simulink model "q"  (R2017b)
settings: Solver=ode5  StartTime=0.0  StopTime=10.0  FixedStep=60  RelTol=1e-3
values from neighbouring files (symbols this model uses):
  AU = 1.496e11    (= 149600000000)    [Dyn_kin.m]    (also in trans_kin_dyn.m)
  c = SC.Polyhedron.C    [Dyn_kin.m]    (also in trans_kin_dyn.m)
  G = 6.674080000000000e-11    (= 6.67408e-11)    [Dyn_kin.m]    (also in trans_kin_dyn.m)
  mu_s = 1.326807104e20    (= 1.326807104e+20)    [Dyn_kin.m]    (also in trans_kin_dyn.m)
  T = [0 2000]    [Att_dyn.m]    (also in Att_kin.m; Dyn_kin.m = [0 1000]; trans_kin_dyn.m = [0 1000])
undefined symbols (not defined in the file or in its folder): bias, Cube, K_d, K_p, noise, P_k0, SC, std_noise, Sun, x_k0
settings Model: Creator=hazr_sh  LastModifiedBy=hazr_sh

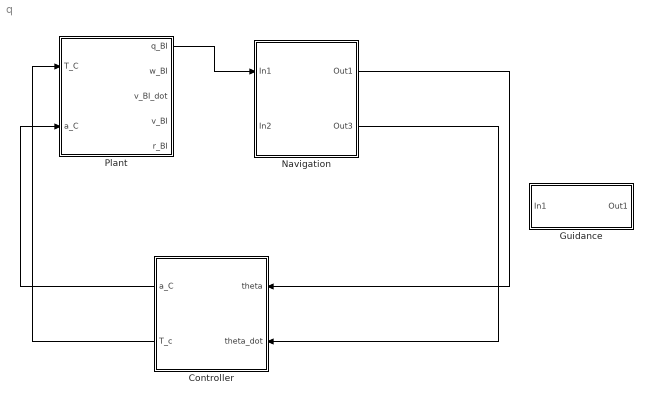
== system q ==
  Controller : Subsystem
  Guidance : Subsystem
  Navigation : Subsystem
  Plant : Subsystem
  wires:
  Controller/2(T_c) -> Plant/1(T_C)
  Plant/1(q_BI) -> Navigation/1(In1)
  ? -> Navigation/2(In2)
  Navigation/1(Out1) -> Controller/1(theta)
  Navigation/2(Out3) -> Controller/2(theta_dot)
  Controller/1(a_C) -> Plant/2(a_C)

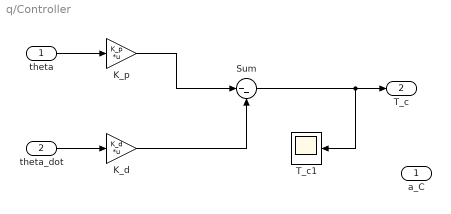
== system q/Controller ==
  theta : Inport
  theta_dot : Inport  Port=2
  K_d : Gain  Gain=K_d  Multiplication=Matrix(K*u)
  K_p : Gain  Gain=K_p  Multiplication=Matrix(K*u)
  Sum : Sum  Inputs=|--
  T_c1 : Scope
  a_C : Outport
  T_c : Outport  Port=2
  wires:
  theta_dot/1 -> K_d/1
  theta/1 -> K_p/1
  K_p/1 -> Sum/1
  K_d/1 -> Sum/2
  Sum/1 -> T_c1/1, T_c/1

== system q/Guidance ==
  In1 : Inport
  Out1 : Outport
  wires:
  In1/1 -> Out1/1

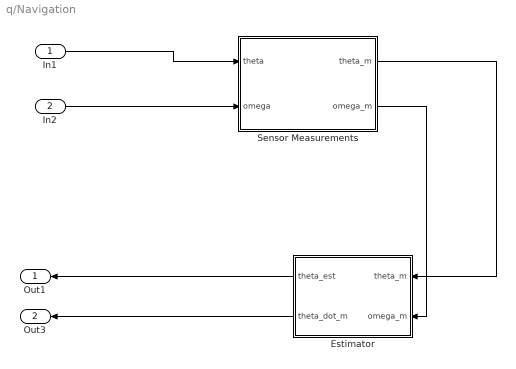
== system q/Navigation ==
  In1 : Inport
  In2 : Inport  Port=2
  Estimator : Subsystem
  Sensor Measurements : Subsystem
  Out1 : Outport
  Out3 : Outport  Port=2
  wires:
  Sensor Measurements/2(omega_m) -> Estimator/2(omega_m)
  In2/1 -> Sensor Measurements/2(omega)
  Estimator/1(theta_est) -> Out1/1
  Estimator/2(theta_dot_m) -> Out3/1
  Sensor Measurements/1(theta_m) -> Estimator/1(theta_m)
  In1/1 -> Sensor Measurements/1(theta)

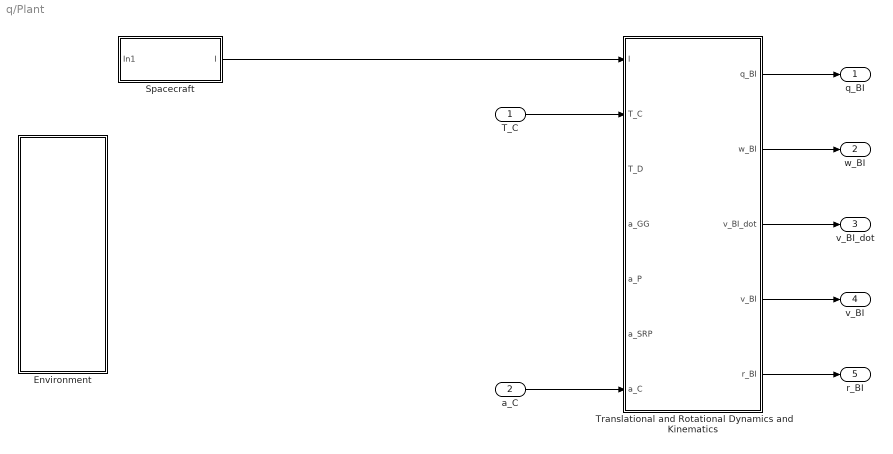
== system q/Plant ==
  T_C : Inport
  a_C : Inport  Port=2
  Environment : Subsystem
  Spacecraft : Subsystem
  Translational and Rotational Dynamics and Kinematics : Subsystem
  q_BI : Outport
  w_BI : Outport  Port=2
  v_BI_dot : Outport  Port=3
  v_BI : Outport  Port=4
  r_BI : Outport  Port=5
  wires:
  Translational and Rotational Dynamics and Kinematics/1(q_BI) -> q_BI/1
  Translational and Rotational Dynamics and Kinematics/2(w_BI) -> w_BI/1
  Translational and Rotational Dynamics and Kinematics/3(v_BI_dot) -> v_BI_dot/1
  Translational and Rotational Dynamics and Kinematics/4(v_BI) -> v_BI/1
  Translational and Rotational Dynamics and Kinematics/5(r_BI) -> r_BI/1
  ? -> Translational and Rotational Dynamics and Kinematics/4(a_GG)
  ? -> Translational and Rotational Dynamics and Kinematics/5(a_P)
  ? -> Translational and Rotational Dynamics and Kinematics/6(a_SRP)
  a_C/1 -> Translational and Rotational Dynamics and Kinematics/7(a_C)
  T_C/1 -> Translational and Rotational Dynamics and Kinematics/2(T_C)
  Spacecraft/1(I) -> Translational and Rotational Dynamics and Kinematics/1(I)
  ? -> Translational and Rotational Dynamics and Kinematics/3(T_D)

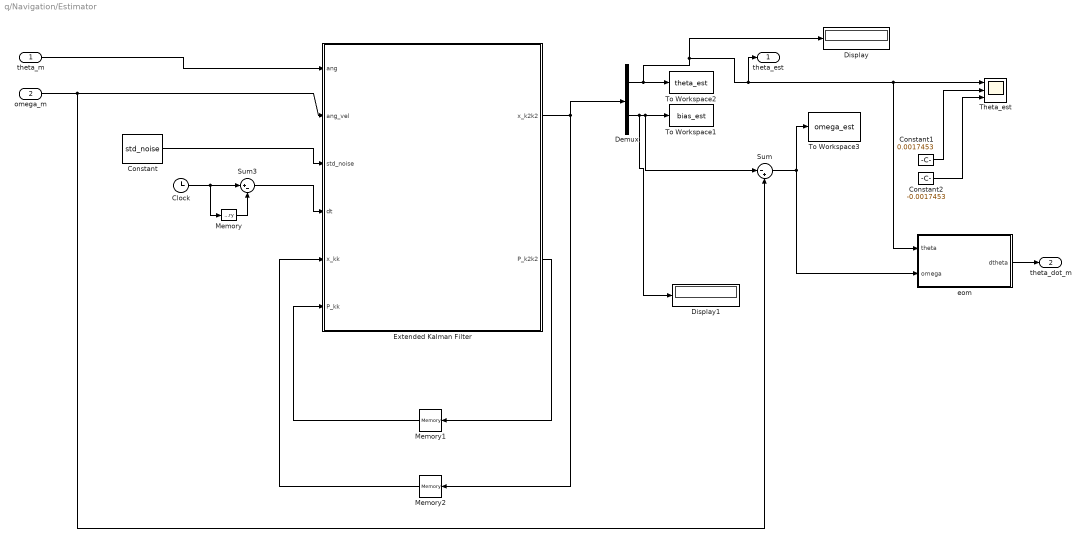
== system q/Navigation/Estimator ==
  theta_m : Inport
  omega_m : Inport  Port=2
  " Extended Kalman Filter" : MATLAB Function  TreatAsAtomicUnit=on
  Clock : Clock
  Constant : Constant  Value=std_noise  VectorParams1D=off
  Constant1 : Constant  Value=0.0017453
  Constant2 : Constant  Value=-0.0017453
  Demux : Demux  Outputs=2
  Display : Display
  Display1 : Display
  Memory : Memory
  Memory1 : Memory  InitialCondition=P_k0
  Memory2 : Memory  InitialCondition=x_k0
  Sum : Sum  Inputs=|-+
  Sum3 : Sum  Inputs=|+-
  Theta_est : Scope  NumInputPorts=3
  To Workspace1 : ToWorkspace  VariableName=bias_est  SampleTime=-1
  To Workspace2 : ToWorkspace  VariableName=theta_est  SampleTime=-1
  To Workspace3 : ToWorkspace  VariableName=omega_est  SampleTime=-1
  "eom " : MATLAB Function  TreatAsAtomicUnit=on
  theta_est : Outport
  theta_dot_m : Outport  Port=2
  wires:
  Memory1/1 -> " Extended Kalman Filter"/6(P_kk)
  theta_m/1 -> " Extended Kalman Filter"/1(ang)
  Memory/1 -> Sum3/2
  Clock/1 -> Memory/1, Sum3/1
  " Extended Kalman Filter"/2(P_k2k2) -> Memory1/1
  " Extended Kalman Filter"/1(x_k2k2) -> Demux/1, Memory2/1
  Sum3/1 -> " Extended Kalman Filter"/4(dt)
  omega_m/1 -> Sum/2, " Extended Kalman Filter"/2(ang_vel)
  Memory2/1 -> " Extended Kalman Filter"/5(x_kk)
  Constant/1 -> " Extended Kalman Filter"/3(std_noise)
  Constant1/1 -> Theta_est/2
  Constant2/1 -> Theta_est/3
  Sum/1 -> To Workspace3/1, "eom "/2(omega)
  "eom "/1(dtheta) -> theta_dot_m/1
  Demux/1 -> To Workspace2/1, theta_est/1, "eom "/1(theta), Theta_est/1, Display/1
  Demux/2 -> Sum/1, To Workspace1/1, Display1/1

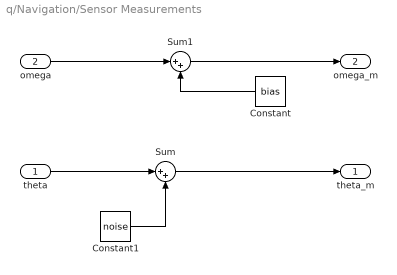
== system q/Navigation/Sensor Measurements ==
  theta : Inport
  omega : Inport  Port=2
  Constant : Constant  Value=bias  VectorParams1D=off
  Constant1 : Constant  Value=noise  VectorParams1D=off
  Sum : Sum  Inputs=|++
  Sum1 : Sum  Inputs=|++
  theta_m : Outport
  omega_m : Outport  Port=2
  wires:
  theta/1 -> Sum/1
  Constant1/1 -> Sum/2
  omega/1 -> Sum1/1
  Constant/1 -> Sum1/2
  Sum/1 -> theta_m/1
  Sum1/1 -> omega_m/1

== system q/Plant/Environment ==
  Asteroid Kinematics and Dynamics : Subsystem
  Disturbances : Subsystem

== system q/Plant/Spacecraft ==
  In1 : Inport
  Switch : Switch  Criteria=u2 > Threshold
  I : Outport
  wires:
  In1/1 -> I/1

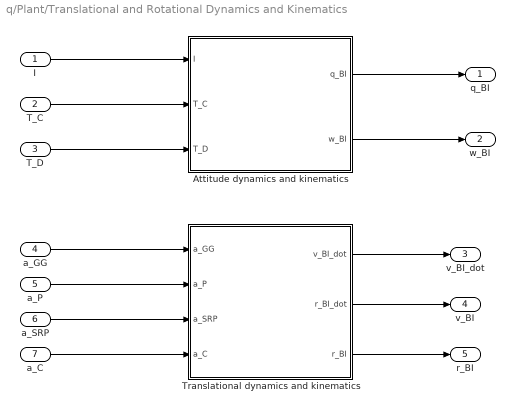
== system q/Plant/Translational and Rotational Dynamics and Kinematics ==
  I : Inport
  T_C : Inport  Port=2
  T_D : Inport  Port=3
  a_GG : Inport  Port=4
  a_P : Inport  Port=5
  a_SRP : Inport  Port=6
  a_C : Inport  Port=7
  Attitude dynamics and kinematics : Subsystem
  Translational dynamics and kinematics : Subsystem
  q_BI : Outport
  w_BI : Outport  Port=2
  v_BI_dot : Outport  Port=3
  v_BI : Outport  Port=4
  r_BI : Outport  Port=5
  wires:
  T_D/1 -> Attitude dynamics and kinematics/3(T_D)
  a_GG/1 -> Translational dynamics and kinematics/1(a_GG)
  a_SRP/1 -> Translational dynamics and kinematics/3(a_SRP)
  a_P/1 -> Translational dynamics and kinematics/2(a_P)
  I/1 -> Attitude dynamics and kinematics/1(I)
  Translational dynamics and kinematics/2(r_BI_dot) -> v_BI/1
  Attitude dynamics and kinematics/1(q_BI) -> q_BI/1
  T_C/1 -> Attitude dynamics and kinematics/2(T_C)
  Translational dynamics and kinematics/3(r_BI) -> r_BI/1
  Translational dynamics and kinematics/1(v_BI_dot) -> v_BI_dot/1
  Attitude dynamics and kinematics/2(w_BI) -> w_BI/1
  a_C/1 -> Translational dynamics and kinematics/4(a_C)

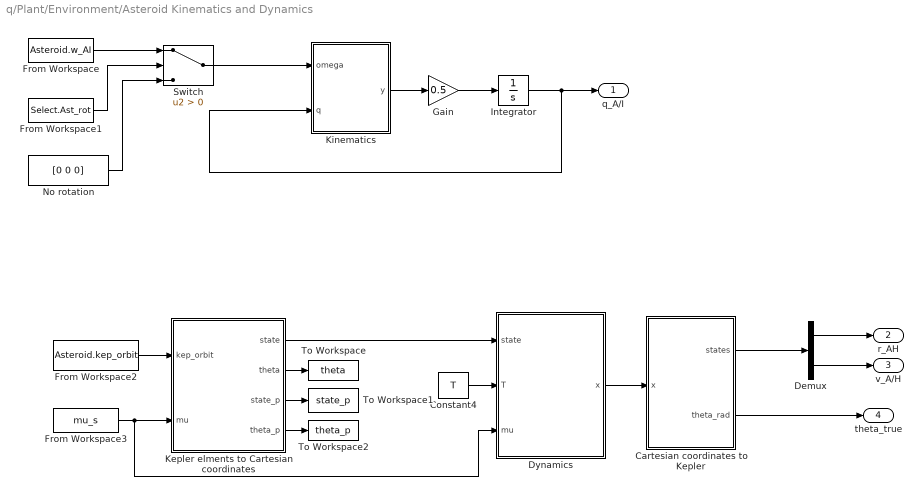
== system q/Plant/Environment/Asteroid Kinematics and Dynamics ==
  Cartesian coordinates to Kepler : MATLAB Function  TreatAsAtomicUnit=on
  Constant4 : Constant  Value=T
  Demux : Demux  Outputs=2
  Dynamics : MATLAB Function  TreatAsAtomicUnit=on
  From Workspace : FromWorkspace  VariableName=Asteroid.w_AI  SampleTime=0
  From Workspace1 : FromWorkspace  VariableName=Select.Ast_rot  SampleTime=0
  From Workspace2 : FromWorkspace  VariableName=Asteroid.kep_orbit  SampleTime=0
  From Workspace3 : FromWorkspace  VariableName=mu_s  SampleTime=0
  Gain : Gain  Gain=0.5
  Integrator : Integrator  InitialCondition=[0 0 0]
  Kepler elments to Cartesian coordinates : MATLAB Function  TreatAsAtomicUnit=on
  Kinematics : MATLAB Function  TreatAsAtomicUnit=on
  No rotation : Constant  Value=[0 0 0]  VectorParams1D=off
  Switch : Switch  Criteria=u2 > Threshold
  To Workspace : ToWorkspace  VariableName=theta  SampleTime=-1
  To Workspace1 : ToWorkspace  VariableName=state_p  SampleTime=-1
  To Workspace2 : ToWorkspace  VariableName=theta_p  SampleTime=-1
  q_A/I : Outport
  r_AH : Outport  Port=2
  v_A/H : Outport  Port=3
  theta_true : Outport  Port=4
  wires:
  Integrator/1 -> Kinematics/2(q), q_A/I/1
  Kinematics/1(y) -> Gain/1
  From Workspace/1 -> Switch/1
  Gain/1 -> Integrator/1
  Switch/1 -> Kinematics/1(omega)
  From Workspace1/1 -> Switch/2
  No rotation/1 -> Switch/3
  Dynamics/1(x) -> Cartesian coordinates to Kepler/1(x)
  Kepler elments to Cartesian coordinates/1(state) -> Dynamics/1(state)
  From Workspace3/1 -> Kepler elments to Cartesian coordinates/2(mu), Dynamics/3(mu)
  Constant4/1 -> Dynamics/2(T)
  Cartesian coordinates to Kepler/1(states) -> Demux/1
  Cartesian coordinates to Kepler/2(theta_rad) -> theta_true/1
  Demux/1 -> r_AH/1
  Demux/2 -> v_A/H/1
  From Workspace2/1 -> Kepler elments to Cartesian coordinates/1(kep_orbit)
  Kepler elments to Cartesian coordinates/2(theta) -> To Workspace/1
  Kepler elments to Cartesian coordinates/3(state_p) -> To Workspace1/1
  Kepler elments to Cartesian coordinates/4(theta_p) -> To Workspace2/1

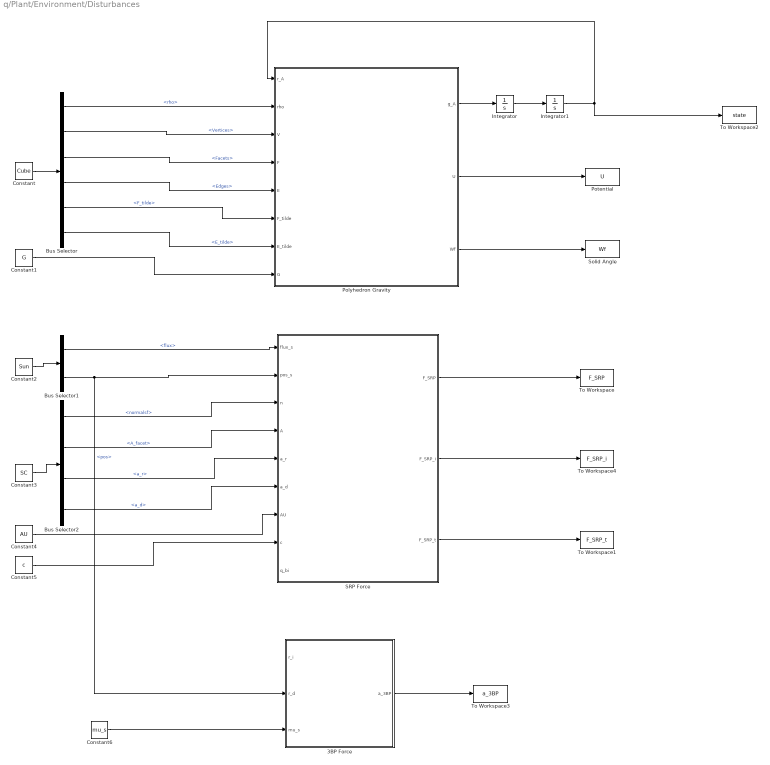
== system q/Plant/Environment/Disturbances ==
  3BP Force : MATLAB Function  TreatAsAtomicUnit=on
  Bus Selector : BusSelector  OutputSignals=rho,Polyhedron.Vertices,Polyhedron.Facets,Polyhedron.Edges,Polyhedron.F_tilde,Polyhedron.E_tilde
  Bus Selector1 : BusSelector  OutputSignals=flux,pos
  Bus Selector2 : BusSelector  OutputSignals=Polyhedron.normalsf,Polyhedron.A_facet,a_r,a_d
  Constant : Constant  Value=Cube  VectorParams1D=off  OutDataTypeStr=Bus: slBus1
  Constant1 : Constant  Value=G
  Constant2 : Constant  Value=Sun  VectorParams1D=off  OutDataTypeStr=Bus: slBus2
  Constant3 : Constant  Value=SC  VectorParams1D=off  OutDataTypeStr=Bus: slBus3
  Constant4 : Constant  Value=AU
  Constant5 : Constant  Value=c
  Constant6 : Constant  Value=mu_s
  Integrator : Integrator  InitialCondition=SC.v_init
  Integrator1 : Integrator  InitialCondition=SC.x_init
  Polyhedron Gravity : MATLAB Function  TreatAsAtomicUnit=on
  Potential : ToWorkspace  VariableName=U  SaveFormat=Timeseries  SampleTime=-1
  SRP Force : MATLAB Function  TreatAsAtomicUnit=on
  Solid Angle : ToWorkspace  VariableName=Wf  SaveFormat=Timeseries  SampleTime=-1
  To Workspace : ToWorkspace  VariableName=F_SRP  SampleTime=-1
      settings: Save2DSignal=2-D array (concatenate along first dimension)
  To Workspace1 : ToWorkspace  VariableName=F_SRP_t  SampleTime=-1
      settings: Save2DSignal=2-D array (concatenate along first dimension)
  To Workspace2 : ToWorkspace  VariableName=state  SampleTime=-1
  To Workspace3 : ToWorkspace  VariableName=a_3BP  SampleTime=-1
      settings: Save2DSignal=2-D array (concatenate along first dimension)
  To Workspace4 : ToWorkspace  VariableName=F_SRP_i  SampleTime=-1
      settings: Save2DSignal=2-D array (concatenate along first dimension)
  wires:
  ? -> SRP Force/9(q_bi)
  ? -> 3BP Force/1(r_i)
  Constant1/1 -> Polyhedron Gravity/8(G)
  Bus Selector/1 -> Polyhedron Gravity/2(rho)  "<rho>"
  Bus Selector/4 -> Polyhedron Gravity/5(E)  "<Edges>"
  Constant/1 -> Bus Selector/1
  Polyhedron Gravity/2(U) -> Potential/1
  Integrator/1 -> Integrator1/1
  SRP Force/3(F_SRP_t) -> To Workspace1/1
  SRP Force/2(F_SRP_i) -> To Workspace4/1
  Integrator1/1 -> To Workspace2/1, Polyhedron Gravity/1(r_A)
  Polyhedron Gravity/1(g_A) -> Integrator/1
  Polyhedron Gravity/3(Wf) -> Solid Angle/1
  Bus Selector2/2 -> SRP Force/4(A)  "<A_facet>"
  Bus Selector1/1 -> SRP Force/1(flux_s)  "<flux>"
  Constant3/1 -> Bus Selector2/1
  Constant5/1 -> SRP Force/8(c)
  Constant6/1 -> 3BP Force/3(mu_s)
  Constant4/1 -> SRP Force/7(AU)
  Bus Selector1/2 -> 3BP Force/2(r_d), SRP Force/2(pos_s)  "<pos>"
  Bus Selector2/1 -> SRP Force/3(n)  "<normalsf>"
  Bus Selector2/3 -> SRP Force/5(a_r)  "<a_r>"
  Bus Selector2/4 -> SRP Force/6(a_d)  "<a_d>"
  Bus Selector/2 -> Polyhedron Gravity/3(V)  "<Vertices>"
  SRP Force/1(F_SRP) -> To Workspace/1
  Bus Selector/6 -> Polyhedron Gravity/7(E_tilde)  "<E_tilde>"
  Bus Selector/3 -> Polyhedron Gravity/4(F)  "<Facets>"
  Bus Selector/5 -> Polyhedron Gravity/6(F_tilde)  "<F_tilde>"
  3BP Force/1(a_3BP) -> To Workspace3/1
  Constant2/1 -> Bus Selector1/1

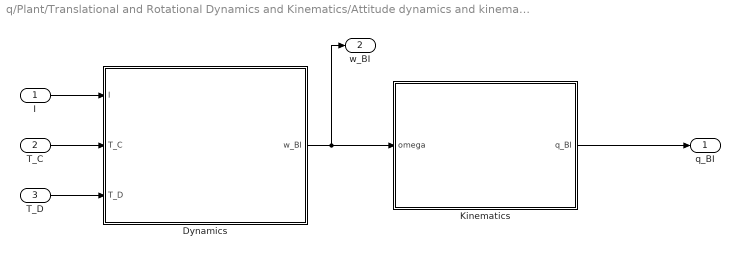
== system q/Plant/Translational and Rotational Dynamics and Kinematics/Attitude dynamics and kinematics ==
  I : Inport
  T_C : Inport  Port=2
  T_D : Inport  Port=3
  Dynamics : Subsystem
  Kinematics : Subsystem
  q_BI : Outport
  w_BI : Outport  Port=2
  wires:
  T_C/1 -> Dynamics/2(T_C)
  Kinematics/1(q_BI) -> q_BI/1
  Dynamics/1(w_BI) -> w_BI/1, Kinematics/1(omega)
  T_D/1 -> Dynamics/3(T_D)
  I/1 -> Dynamics/1(I)

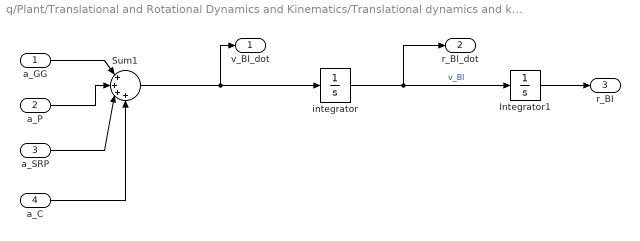
== system q/Plant/Translational and Rotational Dynamics and Kinematics/Translational dynamics and kinematics ==
  a_GG : Inport
  a_P : Inport  Port=2
  a_SRP : Inport  Port=3
  a_C : Inport  Port=4
  " integrator" : Integrator  InitialCondition=[0,0,0]'
  Integrator1 : Integrator  InitialCondition=[0.1745 0.1745 0.1745]'
  Sum1 : Sum  Inputs=|++++
  v_BI_dot : Outport
  r_BI_dot : Outport  Port=2
  r_BI : Outport  Port=3
  wires:
  a_GG/1 -> Sum1/1
  " integrator"/1 -> r_BI_dot/1, Integrator1/1  "v_BI"
  a_P/1 -> Sum1/2
  Sum1/1 -> v_BI_dot/1, " integrator"/1
  Integrator1/1 -> r_BI/1
  a_SRP/1 -> Sum1/3
  a_C/1 -> Sum1/4

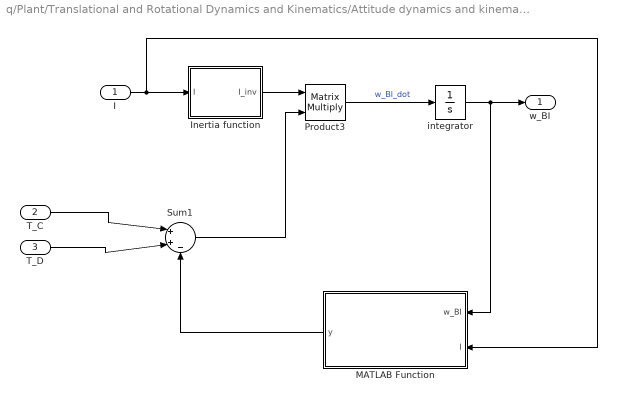
== system q/Plant/Translational and Rotational Dynamics and Kinematics/Attitude dynamics and kinematics/Dynamics ==
  I : Inport
  T_C : Inport  Port=2
  T_D : Inport  Port=3
  " integrator" : Integrator  InitialCondition=[0,0,0]'
  "Inertia function " : MATLAB Function  TreatAsAtomicUnit=on
  MATLAB Function : MATLAB Function  TreatAsAtomicUnit=on
  Product3 : Product  Multiplication=Matrix(*)
  Sum1 : Sum  Inputs=|++-
  w_BI : Outport
  wires:
  Product3/1 -> " integrator"/1  "w_BI_dot"
  T_D/1 -> Sum1/2
  Sum1/1 -> Product3/2
  "Inertia function "/1(I_inv) -> Product3/1
  T_C/1 -> Sum1/1
  " integrator"/1 -> w_BI/1, MATLAB Function/1(w_BI)
  I/1 -> MATLAB Function/2(I), "Inertia function "/1(I)
  MATLAB Function/1(y) -> Sum1/3

== system q/Plant/Translational and Rotational Dynamics and Kinematics/Attitude dynamics and kinematics/Kinematics ==
  omega : Inport
  Gain : Gain  Gain=0.5
  Integrator : Integrator  InitialCondition=[0.1745 0.1745 0.1745]'
  cross_quat : MATLAB Function  TreatAsAtomicUnit=on
  q_BI : Outport
  wires:
  Integrator/1 -> cross_quat/2(p), q_BI/1
  omega/1 -> cross_quat/1(q)
  cross_quat/1(y) -> Gain/1
  Gain/1 -> Integrator/1

== matlab function q/Navigation/Estimator/ Extended Kalman Filter ==
  data: ang input; ang_vel input; std_noise input; dt input; x_kk input; P_kk input; x_k2k2 output; P_k2k2 output; n parameter
function [x_k2k2,P_k2k2] = ekf(ang,ang_vel,std_noise,dt,x_kk,P_kk,n)

%% Current state and measurement vector
theta = [x_kk(1,1) x_kk(2,1) x_kk(3,1)]';
b = [x_kk(4,1) x_kk(5,1) x_kk(6,1)]';
z_k1k1 = ang;

%% Covariance matrices
H = [eye(3) zeros(3,3)];
R = diag((std_noise.^2)'); %measurement noise covariance
Q = 0.*eye(6);           %process noise covariance

%% Jacobian matrix
s1 = sin(theta(1));
s2 = sin(theta(2));
s3 = sin(theta(3));
c1 = cos(theta(1));
c2 = cos(theta(2));
c3 = cos(theta(3));
t2 = s2/c2;

Jf1 = [(b(3)*s1*t2-b(2)*c1*t2) (n*s2*s3/c2^2-b(2)*s1-b(3)*c1*t2^2-b(2)*s1*(t2^2)-b(3)*c1) (n*c3/c2) (-1) -(s1*t2) -(c1*t2)]; 
Jf2 = [(b(3)*c1+b(2)*s1) 0 (-n*s3) 0 -c1 s1];
Jf3 = [(b(3)*s1/c2-b(2)*c1/c2)  (n*s3+n*s3*t2^2-b(3)*c1*s2/c2^2-b(2)*s1*s2/c2^2) (n*c3*t2) 0 -s1/c2 -c1/c2];
Jf4 = zeros(3,6);

J_f = [Jf1;Jf2;Jf3;Jf4];

%% State transition
phi = eye(6) + J_f*dt + 1/2*J_f^2*dt^2;

%State vector dynamics
x_k_dot = der(ang_vel,x_kk,n);

%% Prediction 
x_k2k = x_kk + x_k_dot*dt;
P_k2k = phi*P_kk*phi' + Q;

%% Correction
K_kk = (P_k2k*H')/(H*P_k2k*H'+R); %Kalman gain

%% Update
x_k2k2 = x_k2k + K_kk*(z_k1k1 - H*x_k2k); %measurement update
P_k2k2 = (eye(6) - K_kk*H)*P_k2k*(eye(6) - K_kk*H)' + K_kk*R*K_kk';
end

== matlab function q/Plant/Environment/Asteroid Kinematics and Dynamics/Kinematics ==
  data: omega input; q input; y output
function y = kin(omega, q)
% Quaternion Cross Product
w1 = omega(1);
w2 = omega(2);
w3 = omega(3);

Omega = [0 w3 -w2 w1
         -w3 0 w1 w2
         w2 -w1 0 w3
         -w1 -w2 -w3 0];


y = Omega*q;
end

== matlab function q/Plant/Environment/Asteroid Kinematics and Dynamics/Dynamics ==
  data: state input; T input; x output; mu input
function x  = Propagate_Orbit(state,T,mu)
%Propagate_Orbit( kepler_orbit, state, mu,tspan)
%This function is to propagate the Kepler orbit subject to only gravity 
%tspan = [0 T+7*24*3600]

% T = 2*pi/kepler_orbit(1,7);
% T = 48*3600;

function dx = kepode(t,x)
r = sqrt(x(1)^2 + x(2)^2 + x(3)^2);
dx = [x(5); x(6); x(7); 0; -mu*x(1)/r^3; -mu*x(2)/r^3; -mu*x(3)/r^3; 0];
end

% opts = odeset('Reltol',1e-13,'AbsTol',1e-14,'Stats','on');
% x0 = state;
% [t,x] = ode113(@kepode, tspan, x0, opts);
% plot(t,x)
% legend('x','x''','y','y''','z','z''')
% title('Position and Velocity Components')
tspan = linspace(T.t0,T.tf,T.nsteps);
x0 = state;
x = ode4(@kepode,tspan,x0);

end

== matlab function q/Plant/Translational and Rotational Dynamics and Kinematics/Attitude dynamics and kinematics/Dynamics/MATLAB Function ==
  data: w_BI input; I input; y output
function y = fcn(w_BI,I)

y = cross(w_BI, dot(I,w_BI));

end

== matlab function q/Plant/Environment/Asteroid Kinematics and Dynamics/Cartesian coordinates to Kepler ==
  data: x input; states output; theta_rad output
function [states,theta_rad]  = Cart2kep(x)
%% Cartesian components to Kepler elements
X = [];
R = [];
V = [];
v = [];
H = [];
h = [];
N = [];
n = [];
ee = [];
e = [];
N_xy = [];
theta_rad = [];
theta = [];
p = [];
E_rad = [];
E = [];
M = [];
states = [];

for i = 1:length(x)
    X(i,:) = x(i,1:3);  %state vector
    R(i) = norm(X(i,:));  %magnitude of the X vector

    V(i,:) = x(i,5:7); %velocity vector
    v(i) = norm(V(i,:)); %magnitude of the V vector

    H(i,:) = cross(X(i,:),V(i,:)); %Angular momentum
    h(i) = norm(H(i,:));    %magnitude of the H vector

    s = [0 0 1]';   
    N(i,:) = cross(s,H(i,:));   %Nodal Vector
    n(i) = norm (N(i,:));     %magnitude of the N vector

    ee(i,:) = ((cross(V(i,:),H(i,:))./mu) - X(i,:)./R(i));  %calculating eccentricity vector
    e(i) = norm(ee(i,:));

    N_xy = sqrt (N(1)^2 + N(2)^2);

    theta_rad(i,:) = sign (dot(cross(ee(i,:),X(i,:)),H(i,:))) * acos(dot (X(i,:),ee(i,:))/(R(i)*e(i))); %calculating theta in radians
    theta(i,:) = theta_rad(i,:) * 180/pi;

    p(i,:) = sqrt((1-e(i))/(1+e(i))) * tan(theta_rad(i,:)/2);
    E_rad(i,:) = 2 * atan(p(i,:));
    E(i,:) =  E_rad(i,:) * 180 /pi;  %calculating eccentric anomaly

    M(i,:) = (E_rad(i,:) - e(i) * sin(E_rad(i,:))) * 180 /pi; %calculating mean anomaly
end

states(:,1:3) = X;
states(:,5:7) = V;
states(:,4) = 0;
states(:,8) = 0;
% figure
% hold on
% plot3(x(:,1),x(:,2),x(:,3))
% plot3(0,0,0,'ro')
% axis equal
% title('Orbit of ')
end

== matlab function q/Navigation/Estimator/eom  ==
  data: theta input; dtheta output; omega input; n parameter
function dtheta = ang_rate(theta, omega,n)
%#codegen
 E = [cos(theta(2)) sin(theta(1))*sin(theta(2)) cos(theta(1))*sin(theta(2))
     0 cos(theta(1))*cos(theta(2)) -sin(theta(1))*cos(theta(2))
     0 -sin(theta(1)) cos(theta(1))];
 
 F = [sin(theta(3))
     cos(theta(2))*cos(theta(3))
     sin(theta(2))*sin(theta(3))];
 
 dtheta = ((1/cos(theta(2)))*E)*omega + (n/cos(theta(2)))*F;
end

== matlab function q/Plant/Translational and Rotational Dynamics and Kinematics/Attitude dynamics and kinematics/Dynamics/Inertia function  ==
  data: I_inv output; I input
function I_inv = fcn(I)

I_inv = inv(I);

end

== matlab function q/Plant/Translational and Rotational Dynamics and Kinematics/Attitude dynamics and kinematics/Kinematics/cross_quat ==
  data: q input; y output; p input
function y = cross_quat(q, p)
% Quaternion Cross Product

q4= q(4);
p4= p(4);

q_vect= q(1:3);
p_vect= p(1:3);

y = [q4.*p_vect + p4.*q_vect - cross(q_vect, p_vect); q4*p4 - dot(q_vect,p_vect)];
end

== matlab function q/Plant/Environment/Asteroid Kinematics and Dynamics/Kepler elments to Cartesian coordinates ==
  data: kep_orbit input; state output; theta output; mu input; state_p output; theta_p output
function [state,theta,state_p,theta_p] = Kep2cart(kep_orbit,mu)
%% Kepler  elements  to  Cartesian  components
%NASA,2014  data
% kep_orbit(1,1) = 6787746.891;
% kep_orbit(1,2) = 0.000731104;
% kep_orbit(1,3) = 51.68714486*pi /180;
% kep_orbit(1,4) = 127.5486706*pi /180;
% kep_orbit(1,5) = 74.21987137*pi /180;
% kep_orbit(1,6) = 24.06608426*pi /180;


format  long

Etemp = 0;
deltaE = 1;

while  abs ( deltaE ) > 1e-8 %lower limit for the difference
    E = Etemp + (kep_orbit(1,6)-Etemp + kep_orbit(1,2)*sin (Etemp) ) /(1-kep_orbit(1,2)*cos (Etemp) ) ; %updating E
    deltaE = E-Etemp ; %difference
    Etemp = E; %for next iteration
end

r = kep_orbit(1,1)*(1-kep_orbit(1,2)*cos  (E) );  %position with respect to kepler elements
theta = 2*atan ( sqrt ((1 + kep_orbit(1,2) ) /(1-kep_orbit(1,2) ) )*tan  (E/2) );  %calculating the true anomaly
% true_anomaly = rad2deg(theta);

S = [ ( r*cos  ( theta ) ) 
    ( r*sin  ( theta ) ) ] ; %calculating perifocal co-ordinates

l1 = cos (kep_orbit(1,4))*cos (kep_orbit(1,5))-sin  (kep_orbit(1,4))*sin  (kep_orbit(1,5))*cos ( kep_orbit(1,3) ) ;
l2 =-cos (kep_orbit(1,4))*sin (kep_orbit(1,5))-sin  (kep_orbit(1,4))*cos  (kep_orbit(1,5))*cos ( kep_orbit(1,3) ) ;
m1 = sin (kep_orbit(1,4))*cos (kep_orbit(1,5)) + cos  (kep_orbit(1,4))*sin  (kep_orbit(1,5))*cos ( kep_orbit(1,3) ) ;
m2 =-sin (kep_orbit(1,4))*sin (kep_orbit(1,5)) + cos  (kep_orbit(1,4))*cos  (kep_orbit(1,5))*cos ( kep_orbit(1,3) ) ;
n1 = sin  (kep_orbit(1,5))*sin  ( kep_orbit(1,3) ) ;
n2 = cos (kep_orbit(1,5))*sin  ( kep_orbit(1,3) ) ;

H = sqrt (mu*kep_orbit(1,1)*(1-kep_orbit(1,2) ^2) ) ; %calculating angular momentum

L = [ l1  l2
      m1 m2
      n1 n2 ] ;

X = L*S ;  %calculating the state vector
V = [ (mu/H*(-l1*sin  ( theta ) + l2*( kep_orbit(1,2) + cos ( theta ) ) ) )    %calculating the velocity vector
      (mu/H*(-m1*sin  ( theta ) + m2*( kep_orbit(1,2) + cos ( theta ) ) ) )
      (mu/H*(-n1*sin  ( theta ) + n2*( kep_orbit(1,2) + cos ( theta ) ) ) ) ] ;
  
state = [X;0;V;0];
Cartesian = { 'x ' ;  'y ' ;  ' z ' ;  ' xdot ' ;  ' ydot ' ;  ' zdot ' };
Values = [X(1) ; X(2) ; X(3) ; V(1) ; V(2) ; V(3) ] ;
T = table ( Cartesian ,  Values );


%% State at pericentre

format  long
E_p=0;

r_p = kep_orbit(1,1)*(1-kep_orbit(1,2)*cos  (E_p) );  %position with respect to kepler elements
theta_p = 2*atan ( sqrt ((1 + kep_orbit(1,2) ) /(1-kep_orbit(1,2) ) )*tan  (E_p/2) );  %calculating the true anomaly
% true_anomaly_p = rad2deg(theta_p);

S_p = [ ( r_p*cos  ( theta_p ) ) 
    ( r_p*sin  ( theta_p ) ) ] ; %calculating perifocal co-ordinates

l1_p = cos (kep_orbit(1,4))*cos (kep_orbit(1,5))-sin  (kep_orbit(1,4))*sin  (kep_orbit(1,5))*cos ( kep_orbit(1,3) ) ;
l2_p =-cos (kep_orbit(1,4))*sin (kep_orbit(1,5))-sin  (kep_orbit(1,4))*cos  (kep_orbit(1,5))*cos ( kep_orbit(1,3) ) ;
m1_p = sin (kep_orbit(1,4))*cos (kep_orbit(1,5)) + cos  (kep_orbit(1,4))*sin  (kep_orbit(1,5))*cos ( kep_orbit(1,3) ) ;
m2_p =-sin (kep_orbit(1,4))*sin (kep_orbit(1,5)) + cos  (kep_orbit(1,4))*cos  (kep_orbit(1,5))*cos ( kep_orbit(1,3) ) ;
n1_p = sin  (kep_orbit(1,5))*sin  ( kep_orbit(1,3) ) ;
n2_p = cos (kep_orbit(1,5))*sin  ( kep_orbit(1,3) ) ;

H_p = sqrt (mu*kep_orbit(1,1)*(1-kep_orbit(1,2) ^2) ) ; %calculating angular momentum

L_p = [ l1_p  l2_p
      m1_p m2_p
      n1_p n2_p ] ;

X_p = L_p*S_p ;  %calculating the state vector
V_p = [ (mu/H_p*(-l1_p*sin  ( theta_p ) + l2_p*( kep_orbit(1,2) + cos ( theta_p ) ) ) )    %calculating the velocity vector
      (mu/H_p*(-m1_p*sin  ( theta_p ) + m2_p*( kep_orbit(1,2) + cos ( theta_p ) ) ) )
      (mu/H_p*(-n1_p*sin  ( theta_p ) + n2_p*( kep_orbit(1,2) + cos ( theta_p ) ) ) ) ] ;
  
state_p = [X_p;0;V_p;0];

end

== matlab function q/Plant/Environment/Disturbances/3BP Force ==
  data: r_i input; a_3BP output; r_d input; mu_s input
function a_3BP  = F_3BP(r_i,r_d,mu_s)

r_id = norm(r_d - r_i);
a_3BP = -G*m_s*(r_d-r_i/r_id^3 - r_d/norm(r_d)^3); 

end

== matlab function q/Plant/Environment/Disturbances/Polyhedron Gravity ==
  data: r_A input; rho input; V input; F input; E input; F_tilde input; E_tilde input; g_A output; G input; U output; Wf output
function [g_A, U, Wf] = Poly_gravity(r_A,rho,V,F,E,F_tilde,E_tilde,G)
%% Function to calculate Cube gravity from Asteroid structure (from Get_Asteroid function)
%
% Inputs: r_A - position of a field point in Asteroid frame
%         Asteroid - Asteroid structure
%
% Outputs: g_A - gravitational acceleration in Asteroid frame
%          U - gravitational potential in Asteroid frame
%          Wf - THE solid angle, which shows whether the point is in or out
%               It can be used for stopping simulation if SC crashes

%% Initialization

Wf = 0;

Facets = [0 0 0]';
Edges = [0 0 0]';

U_edg = 0;
U_fac = 0;

S = r_A;

for j=1:1:size(E,1)
    
    % Calculate gravity due to edge potential
    
    R1 = V(E(j,1),:);    
    R2 = V(E(j,2),:);    

    Ri = R1'-S;
    ri = norm(Ri);
    
    Rj = R2'-S;
    rj = norm(Rj);
        
    Rij = Rj-Ri;
    eij = norm(Rij);

    Re1 =(Ri+Rj)/2;
   
    Le = log((ri+rj+eij)/(ri+rj-eij));
    
    if Le == Inf
     
        Le = 0;
     
    end
    
    Edges = (Le*E_tilde(:,:,j)*Re1)+Edges;
    U_edg = (Le*Re1'*E_tilde(:,:,j)*Re1)+U_edg;
    
end

 for i=1:1:(size(F,1))
    
    % Calculate gravity due to face potential
    
    R1 = V(F(i,1),:);    
    R2 = V(F(i,2),:);    
    R3 = V(F(i,3),:);
    

    Ri = R1'-S;
    ri = norm(Ri);
    
    Rj = R2'-S;
    rj = norm(Rj);
    
    Rk = R3'-S;
    rk = norm(Rk);
    
    
    wf = 2*atan2(dot(Ri, cross(Rj,Rk)),(ri*rj*rk+ri*dot(Rj,Rk)+rj*dot(Rk,Ri)+rk*dot(Ri,Rj)));
    
    Rf =(Ri+Rj+Rk)/3;

    U_fac = wf*Rf'*F_tilde(:,:,i)*Rf+U_fac;
    Facets = wf*F_tilde(:,:,i)*Rf+Facets;
    
    Wf = wf+Wf;
  
 end

g_A = G*rho*(-Edges+Facets);

U = 0.5*G*rho*(U_edg-U_fac);

end

== matlab function q/Plant/Environment/Disturbances/SRP Force ==
  data: flux_s input; pos_s input; n input; A input; a_r input; a_d input; AU input; c input; F_SRP output; F_SRP_i output; F_SRP_t output; q_bi input
function [F_SRP,F_SRP_i,F_SRP_t]   = F_SRP(flux_s,pos_s,n,A,a_r,a_d,AU,c,q_bi)

e = pos_s(1,1:3)/norm(pos_s(1,1:3));
P = flux_s/(norm(pos_s(1,1:3)/AU)^2*c);

F_SRP = zeros(size(n,1),3); 
for i=1:1:size(n,1)
    
    co = dot(n(i,1:3),e(1,1:3),2);

    if i<=12
        F = -P*A(i,:)*co.*((2*(a_d(1,1)/3 + a_r(1,1)*co))'.*n(i,1:3) + (1-a_r(1,1))'.*e);
        F_SRP(i,:) = F;
    else
        F = -P*A(i,:)*co.*((2*(a_d(1,2)/3 + a_r(1,2)*co))'.*n(i,1:3) + (1-a_r(1,2))'.*e);
        F_SRP(i,:) = F;
    end
    
    
end
% 
F_SRP_i = cross_quat(q_bi,cross_quat([F_SRP 0]',conj_quat(q_bi)));
F_SRP_t = sum(F_SRP);

end
